simulink model "PerfectActuators"  (R2019b)
settings: Solver=FixedStepAuto  StartTime=0.0  StopTime=10.0  MinStep=dT  RelTol=1e-3
settings Model: Creator=asmialek  LastModifiedBy=asmialek

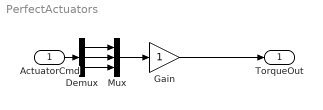
== system PerfectActuators ==
  ActuatorCmd : Inport
  Demux : Demux  Outputs=3
  Gain : Gain
  Mux : Mux  Inputs=3
  TorqueOut : Outport
  wires:
  Gain/1 -> TorqueOut/1
  Demux/1 -> Mux/1
  Demux/2 -> Mux/2
  Demux/3 -> Mux/3
  ActuatorCmd/1 -> Demux/1
  Mux/1 -> Gain/1
